simulink model "ModelProva1"  (R2023a)
settings: Solver=VariableStepAuto  StartTime=0.0  StopTime=10.0  RelTol=1e-3
values from neighbouring files (symbols this model uses):
  A = [0 1 0 0 ... (first row only)    [MainForce.m]    (also in Prova1.m = [ 0 1 0 0)
  A_lift = 3    [MainForce.m]
  AO = A-KO*C    [MainForce.m]
  B1 = [0;0;0;0]    [MainForce.m]
  B2 = [0 0 0 0 0 0 ... (first row only)    [MainForce.m]
  BO = B1-KO*D1    [MainForce.m]
  C = [1 0 0 0 0 ... (first row only)    [MainForce.m]    (also in Prova1.m = [1 0 0 0)
  Cd_lift = 0.5    [MainForce.m]
  Ce = [1 0 0 0 0]    [MainForce.m]
  CO = eye(n)    [MainForce.m]
  D1 = [0;0;0]    [MainForce.m]
  D2 = [0 0 1 0 0 0 ... (first row only)    [MainForce.m]
  De1 = [0]    [MainForce.m]
  De2 = [0 0 1 0 0 -1]    [MainForce.m]
  DT = 1e-4    (= 0.0001)    [MainForce.m]
  e0 = y0(1) - r0    [MainForce.m]
  KI = K(:,n+1:n+m)    [MainForce.m]
  KO = Km.'    [MainForce.m]
  KS = K(:,1:n)    [MainForce.m]
  m = 1    [MainForce.m]
  n = 5    [MainForce.m]
  p = 1    [MainForce.m]
  q = 3    [MainForce.m]
  r = nd + q + m    (= 6)    [MainForce.m]
  r0 = l0s-g*ms/ks    (= 0.64114)    [MainForce.m]
  rho_lift = 1.225    [MainForce.m]
  u0 = 0    [MainForce.m]
  v = 10    [MainForce.m]
  w0 = [d0; nu0; r0]    [MainForce.m]
  x0 = [l0s-g*ms/ks ... (first row only)    [MainForce.m]
  x_init = [zs_init-zu_init ... (first row only)    [MainForce.m]
  x_tilde_init = x_init - x0    [MainForce.m]
  y0 = [x0(1) ... (first row only)    [MainForce.m]
libraries: simulink x3
settings Model: Creator=loreb  LastModifiedBy=loreb

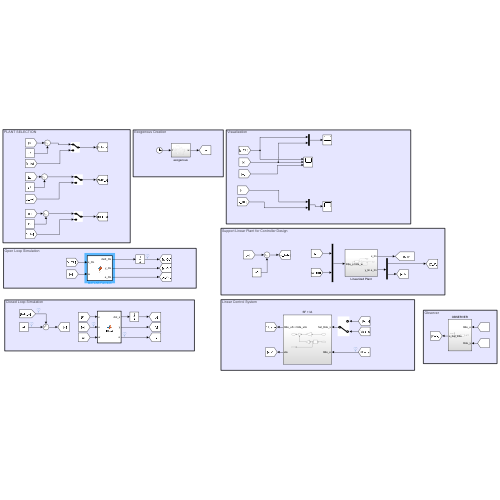
[thumbnail: Simulink's stored preview of the top-level diagram]
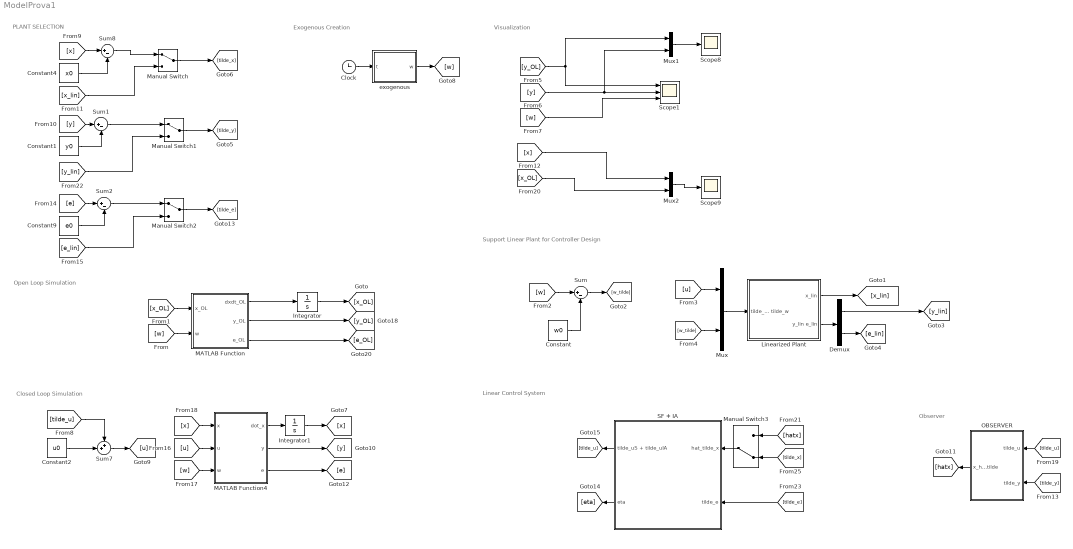
== system ModelProva1 ==
  note: Observer
  note: Open Loop Simulation
  note: Support Linear Plant for Controller Design
  note: Visualization
  note: Exogenous Creation
  note: Closed Loop Simulation
  note: Linear Control System
  note: PLANT SELECTION
  Clock : Clock
  Constant : Constant  Value=w0
  Constant1 : Constant  Value=y0
  Constant2 : Constant  Value=u0
  Constant4 : Constant  Value=x0
  Constant9 : Constant  Value=e0
  Demux : Demux  Outputs=[q m]
  Integrator : Integrator  InitialCondition=x_init
  Integrator1 : Integrator  InitialCondition=x_init
  Linearized Plant : Subsystem
  MATLAB Function : MATLAB Function  TreatAsAtomicUnit=on
  MATLAB Function4 : MATLAB Function  TreatAsAtomicUnit=on
  Manual Switch : ManualSwitch
  Manual Switch1 : ManualSwitch
  Manual Switch2 : ManualSwitch
  Manual Switch3 : ManualSwitch  CurrentSetting=0
  Mux : Mux  Inputs=2
  Mux1 : Mux  Inputs=2
  Mux2 : Mux  Inputs=2
  OBSERVER : Subsystem
  SF + IA : Subsystem
  Scope1 : Scope  NumInputPorts=3
  Scope8 : Scope
  Scope9 : Scope
  Sum{,1..2,8} (4 alike) : Sum  Inputs=|+-
  Sum7 : Sum  Inputs=++|
  exogenous : Subsystem
  wires:
  [x_lin] -> Manual Switch/2
  Manual Switch/1 -> [tilde_x]
  [x] -> Mux2/1
  [tilde_x] -> Manual Switch3/2
  Integrator1/1 -> [x]
  [e_lin] -> Manual Switch2/2
  [x_OL] -> Mux2/2
  [x] -> Sum8/1
  SF + IA/2(eta) -> [eta]
  [w] -> Sum/1
  Manual Switch2/1 -> [tilde_e]
  Sum7/1 -> [u]
  [w_tilde] -> Mux/2
  Sum1/1 -> Manual Switch1/1
  [y_OL] -> Mux1/1, Scope1/1
  Constant9/1 -> Sum2/2
  Manual Switch3/1 -> SF + IA/1(hat_tilde_x)
  MATLAB Function4/2(y) -> [y]
  [tilde_u] -> OBSERVER/1(tilde_u)
  [w] -> Scope1/3
  Sum2/1 -> Manual Switch2/1
  Mux1/1 -> Scope8/1
  Linearized Plant/2(y_lin e_lin) -> Demux/1
  Sum/1 -> [w_tilde]
  Constant4/1 -> Sum8/2
  Sum8/1 -> Manual Switch/1
  [y] -> Sum1/1
  [tilde_y] -> OBSERVER/2(tilde_y)
  [tilde_e] -> SF + IA/2(tilde_e)
  OBSERVER/1(x_hat_tilde) -> [hatx]
  MATLAB Function/2(y_OL) -> [y_OL]
  Manual Switch1/1 -> [tilde_y]
  [e] -> Sum2/1
  [hatx] -> Manual Switch3/1
  MATLAB Function/1(dxdt_OL) -> Integrator/1
  MATLAB Function/3(e_OL) -> [e_OL]
  MATLAB Function4/3(e) -> [e]
  [y_lin] -> Manual Switch1/2
  SF + IA/1(tilde_uS + tilde_uIA) -> [tilde_u]
  [y] -> Mux1/2, Scope1/2
  [w] -> MATLAB Function/2(w)
  [tilde_u] -> Sum7/1
  [u] -> Mux/1
  Demux/1 -> [y_lin]
  [w] -> MATLAB Function4/3(w)
  Constant/1 -> Sum/2
  [u] -> MATLAB Function4/2(u)
  Mux2/1 -> Scope9/1
  exogenous/1(w) -> [w]
  Integrator/1 -> [x_OL]
  MATLAB Function4/1(dot_x) -> Integrator1/1
  Constant2/1 -> Sum7/2
  Constant1/1 -> Sum1/2
  Linearized Plant/1(x_lin) -> [x_lin]
  Demux/2 -> [e_lin]
  Clock/1 -> exogenous/1(t)
  Mux/1 -> Linearized Plant/1(tilde_u tilde_w)
  [x_OL] -> MATLAB Function/1(x_OL)
  [x] -> MATLAB Function4/1(x)

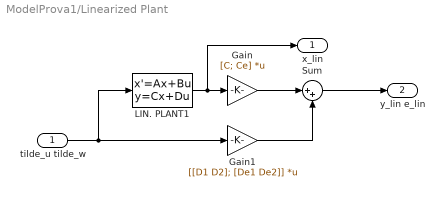
== system ModelProva1/Linearized Plant ==
  tilde_u tilde_w : Inport
  Gain : Gain  Gain=[C; Ce]  Multiplication=Matrix(K*u)
  Gain1 : Gain  Gain=[[D1 D2]; [De1 De2]]  Multiplication=Matrix(K*u)
  LIN. PLANT1 : StateSpace  A=A  B=[B1 B2]  C=eye(n)  D=zeros(n,p+r)  InitialCondition=x_tilde_init  ParameterTunability=Unconstrained
  Sum : Sum  Inputs=|++
  x_lin : Outport
  y_lin e_lin : Outport  Port=2
  wires:
  LIN. PLANT1/1 -> x_lin/1, Gain/1
  tilde_u tilde_w/1 -> LIN. PLANT1/1, Gain1/1
  Gain1/1 -> Sum/2
  Gain/1 -> Sum/1
  Sum/1 -> y_lin e_lin/1

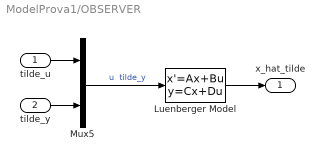
== system ModelProva1/OBSERVER ==
  tilde_u : Inport
  tilde_y : Inport  Port=2
  Luenberger Model : StateSpace  A=AO  B=[BO KO]  C=CO  D=zeros(n,p+q)  InitialCondition=x_tilde_init
  Mux5 : Mux  Inputs=2
  x_hat_tilde : Outport
  wires:
  tilde_u/1 -> Mux5/1
  Mux5/1 -> Luenberger Model/1  "u  tilde_y"
  tilde_y/1 -> Mux5/2
  Luenberger Model/1 -> x_hat_tilde/1

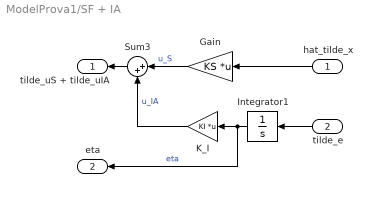
== system ModelProva1/SF + IA ==
  hat_tilde_x : Inport
  tilde_e : Inport  Port=2
  Gain : Gain  Gain=KS  Multiplication=Matrix(K*u)
  Integrator1 : Integrator
  K_I : Gain  Gain=KI  Multiplication=Matrix(K*u)
  Sum3 : Sum  Inputs=|++
  tilde_uS + tilde_uIA : Outport
  eta : Outport  Port=2
  wires:
  Gain/1 -> Sum3/1  "u_S"
  Integrator1/1 -> eta/1, K_I/1  "eta"
  tilde_e/1 -> Integrator1/1
  K_I/1 -> Sum3/2  "u_IA"
  hat_tilde_x/1 -> Gain/1
  Sum3/1 -> tilde_uS + tilde_uIA/1

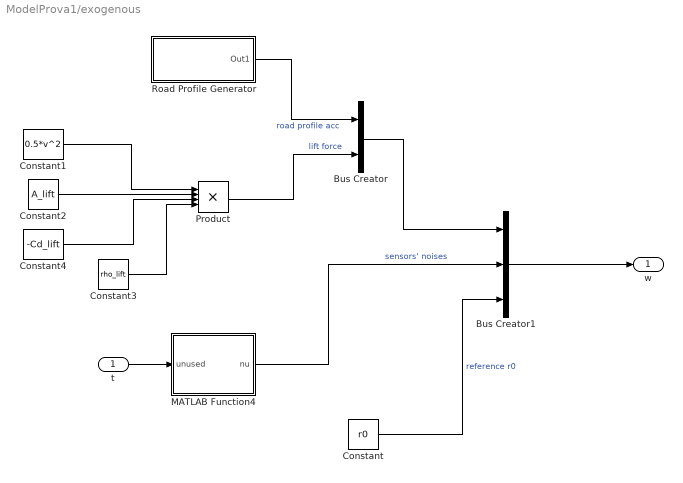
== system ModelProva1/exogenous ==
  t : Inport
  Bus Creator : BusCreator  Inputs=2
  Bus Creator1 : BusCreator  Inputs=3
  Constant : Constant  Value=r0
  Constant1 : Constant  Value=0.5*v^2  SampleTime=DT
  Constant2 : Constant  Value=A_lift  SampleTime=DT
  Constant3 : Constant  Value=rho_lift  SampleTime=DT
  Constant4 : Constant  Value=-Cd_lift  SampleTime=DT
  MATLAB Function4 : MATLAB Function  TreatAsAtomicUnit=on  SystemSampleTime=DT
  Product : Product  Inputs=4
  Road Profile Generator : Subsystem
  w : Outport
  wires:
  Constant1/1 -> Product/1
  Road Profile Generator/1(Out1) -> Bus Creator/1  "road profile acc"
  Constant2/1 -> Product/2
  t/1 -> MATLAB Function4/1(unused)
  Constant3/1 -> Product/4
  Constant4/1 -> Product/3
  Product/1 -> Bus Creator/2  "lift force"
  Bus Creator/1 -> Bus Creator1/1
  MATLAB Function4/1(nu) -> Bus Creator1/2  "sensors' noises"
  Constant/1 -> Bus Creator1/3  "reference r0"
  Bus Creator1/1 -> w/1

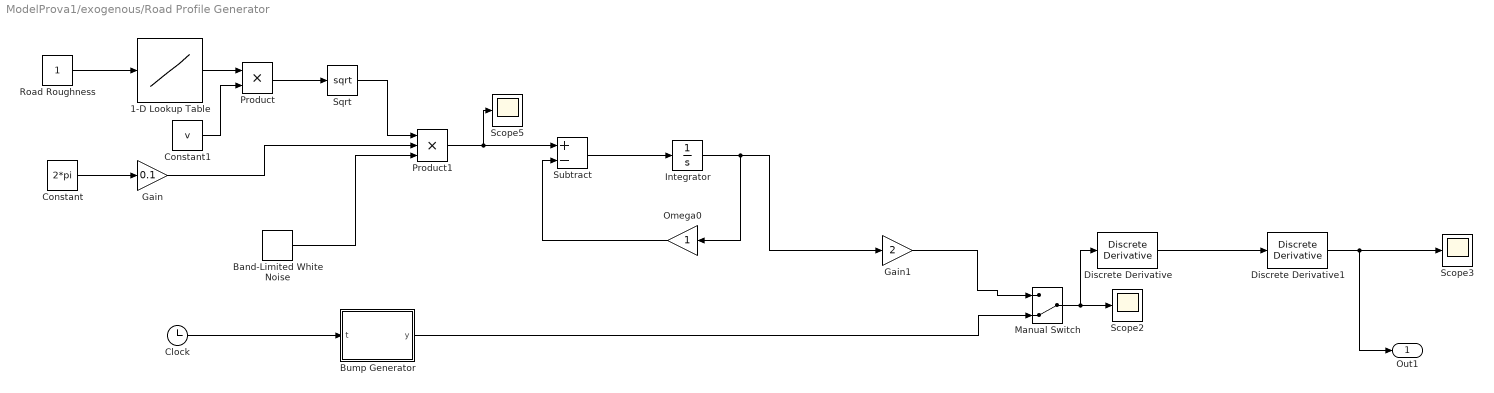
== system ModelProva1/exogenous/Road Profile Generator ==
  1-D Lookup Table : Lookup_n-D  NumberOfTableDimensions=1  BreakpointsForDimension1=[1;2;3;4;5;6;7;8]  Table=[1.6e-05;6.4e-05;0.000256;0.001024;0.004096;0.016384;0.065536;0.262144]  InternalRulePriority=Speed  RndMeth=Simplest
  Band-Limited White Noise : simulink/Sources/Band-Limited White Noise  Cov=0.1  Ts=0.01  seed=[23341]
  Bump Generator : MATLAB Function  TreatAsAtomicUnit=on
  Clock : Clock
  Constant : Constant  Value=2*pi
  Constant1 : Constant  Value=v
  Discrete Derivative : simulink/Quick Insert/Discrete/Discrete Derivative  gainval=1.0  ICPrevScaledInput=0.0  OutMin=[]  OutMax=[]  OutDataType=fixdt(1, 16)  OutScaling=2^-10  DoSatur=off
  Discrete Derivative1 : simulink/Quick Insert/Discrete/Discrete Derivative  gainval=1.0  ICPrevScaledInput=0.0  OutMin=[]  OutMax=[]  OutDataType=fixdt(1, 16)  OutScaling=2^-10  DoSatur=off
  Gain : Gain  Gain=0.1
  Gain1 : Gain  Gain=2
  Integrator : Integrator
  Manual Switch : ManualSwitch  CurrentSetting=0
  Omega0 : Gain
  Product : Product
  Product1 : Product  Inputs=3
  Road Roughness : Constant
  Scope2 : Scope
  Scope3 : Scope
  Scope5 : Scope
  Sqrt : Sqrt
  Subtract : Sum  Inputs=+-
  Out1 : Outport
  wires:
  Subtract/1 -> Integrator/1
  Road Roughness/1 -> 1-D Lookup Table/1
  Clock/1 -> Bump Generator/1(t)
  1-D Lookup Table/1 -> Product/1
  Sqrt/1 -> Product1/1
  Constant/1 -> Gain/1
  Band-Limited White Noise/1 -> Product1/3
  Omega0/1 -> Subtract/2
  Bump Generator/1(y) -> Manual Switch/2
  Product1/1 -> Scope5/1, Subtract/1
  Integrator/1 -> Omega0/1, Gain1/1
  Constant1/1 -> Product/2
  Product/1 -> Sqrt/1
  Gain/1 -> Product1/2
  ? -> ?
  Gain1/1 -> Manual Switch/1
  Discrete Derivative/1 -> Discrete Derivative1/1
  Discrete Derivative1/1 -> Out1/1, Scope3/1
  Manual Switch/1 -> Scope2/1, Discrete Derivative/1

== matlab function ModelProva1/MATLAB Function ==
  data: dxdt_OL output; x_OL input; y_OL output; w input; e_OL output
function [dxdt_OL, y_OL, e_OL] = f(x_OL,w)

x1 = x_OL(1);
x2 = x_OL(2);
x3 = x_OL(3);
x4 = x_OL(4);
x5 = x_OL(5);

% Disturbance
d=w(1);
Lift = w(2);

% Noise
ni1 = w(3);
ni2 = w(4);
ni3 = w(5);

% Reference
r0 = w(6);

%% Physical parameters

ms = 300;    % kg
mu = 60;     % kg
bs = 1000;   % N/m/s
ks = 16000 ; % N/m
kt = 190000; % N/m

%% STATE DYNAMICS

% zr is the road height

dxdt1= x2;
dxdt2= -1/ms*(ks*(x1-x3)-bs*(x2-x4) - 1e3*fs;
dxdt3= x4;
dxdt4= -1/mu* (ks*(x1-x3) + bs(x2-x4) - kt(x3-zr) - 1e3*fs);
dxdt5= 0;

dxdt_OL = [dxdt1;dxdt2;dxdt3;dxdt4;dxdt5];

y_OL = [x1+ni1 
     x1+x3+ni2 
     1/ms*(Lift-ms*g-ks*(x1-l0s)-betas*x2)+ni3];

e_OL = x1 + ni1 -r0;

end

== matlab function ModelProva1/exogenous/Road Profile Generator/Bump Generator ==
  data: t input; y output
function y = fcn(t)

% Parameters definition

v = 10; % [m/s] speed of the vehicle

p = v*t; % [m] position that varies with time

pg = 20; % [m] pg is the position of the BEGINNING of the bump

l = 1; % [m] lenght of the hole/bump
h = 0.2; % [m] thickness of the hole/bump

lmat = [l^4 l^5 l^6 l^7 l^8; (l/2)^4 (l/2)^5 (l/2)^6 (l/2)^7 (l/2)^8; 4*l^3 5*l^4 6*l^5 7*l^6 8*l^7; 12*l^2 20*l^3 30*l^4 42*l^5 56*l^6; 24*l 60*l^2 120*l^3 210*l^4 336*l^5;];
lmatinv = inv(lmat);

cmat = zeros(5,1);
hmat = [0 h 0 0 0]';

cmat = lmatinv * hmat;

% Road profile function

if (p>pg && p-pg < l)
    sum = 0;
    for i = 0:8
        if i > 3
            sum = sum + cmat(i-3)*(p-pg)^(i);
        end
    end
    y = sum;
else
    y = 0;
end

== matlab function ModelProva1/exogenous/MATLAB Function4 ==
  data: unused input; nu output
function nu = noises(~)

% definition of the standard deviations of our sensors

std_pot = 0.001; % [m] potentiomenter standard deviation
std_laser = 0.001; %standard deviation laser
std_acc = 110e-6*sqrt(200); % [m/s^2] accelerometer standard deviation

nu = [std_pot*(2*rand(1)-1)
      std_laser*(2*rand(1)-1)
      std_acc*(2*rand(1)-1)];

end

== matlab function ModelProva1/MATLAB Function4 ==
  data: x input; u input; dot_x output; w input; y output; e output
function [dot_x,y,e] = Plant(x,u,w)

x1 = x(1);
x2 = x(2);
x3 = x(3);
x4 = x(4);
x5 = x(5);

% Disturbance
d = w(1);
Lift = w(2);

% Noise
ni1 = w(3);
ni2 = w(4);
ni3 = w(5);

% Reference
r0 = w(6);

%% Plant Parameters
ks = 50000; %spring coefficient
mu = 100;
ms = 300;
l0s = 0.7; % [m] lenght of the sprung for which the force is 0
g = 9.81;
betas = 500; % damping coefficient 

%% STATE DYNAMICS

barm = (mu+ms)/ms;

dotx1 = x2;
dotx2 = barm/mu*(-ks*(x1-l0s)-betas*x2) - 1/mu*ft(x3) + Lift/ms + (barm/mu)*x5;
dotx3 = x4;
dotx4 = -g + ks/mu*(x1-l0s) + betas/mu*x2 + 1/mu*ft(x3) - 1/mu*x5 - d;
dotx5 = u(1);

dot_x = [dotx1;dotx2;dotx3;dotx4;dotx5];


y = [x(1) + ni1 
     x(1) + x(3) + ni2 
     1/ms*(Lift-ms*g-ks*(x1-l0s) - betas*x2 + x5) + ni3];

e = x1 + ni1 - r0;
end


%% SUPPORT FUNCTIONS

% this function allows to diffenciate the linear plant with the non linear
% one, in this case the tire cannot pull the car (physically acceptable)
% in the linear case the tire would pull the car back on the ground (non
% physically acceptable), this is ok if we stay near the equilibrium point

function f = ft(s)
l0t = 0.35; % [m]
kt = 500000; %tyre elastic coefficient
if s > l0t
    f = 0;
else
    f = -kt*(s-l0t);
end
end
